simulink model "Dfig"  (R2017b)
settings: Solver=ode45  StartTime=0.0  StopTime=20  RelTol=1e-3  EnableMultiTasking=on
undefined symbols (not defined in the file): Cbus, D, DiscIntNeverNeededParam, f, Fs, fsw, J, ki_id, ki_n, kp_id, kp_n, Lg, Lm, Lr, Ls, Lsi, p, Ps, Rg, Rr, Rs, sigma, Tem, Ts, Vbus, Vs
libraries: powerlib x15, powerlib_meascontrol x2
settings Model: Creator=admin  LastModifiedBy=admin
settings DataIOCC: LimitDataPoints=on  SaveFormat=Array
settings OptimizationCC: LifeSpan=inf
settings DebuggingCC: UnderspecifiedInitializationDetection=Classic  MergeDetectMultiDrivingBlocksExec=none  SolverPrmCheckMsg=warning  StateNameClashWarn=warning  SFUnexpectedBacktrackingDiag=warning  SFNoUnconditionalDefaultTransitionDiag=warning  SFExecutionAtInitializationDiag=none
settings HardwareCC: ProdBitPerPointer=32  ProdBitPerSizeT=32  ProdBitPerPtrDiffT=32  ProdLargestAtomicFloat=None  ProdIntDivRoundTo=Undefined  ProdEndianess=Unspecified  ProdWordSize=32  ProdHWDeviceType=32-bit Generic
settings ModelReferenceCC: PropagateSignalLabelsOutOfModel=off
settings CodeAppCC: StateflowObjectComments=on
settings GRTTargetCC: TargetLangStandard=C89/C90 (ANSI)  GeneratePreprocessorConditionals=Disable all
settings ConfigComp: CovMetricSettings=dw  CovHtmlReporting=on  CovSaveCumulativeToWorkspaceVar=on  CovSaveSingleToWorkspaceVar=on  CovExternalEMLEnable=off
settings SimscapeCC: SimscapeNormalizeSystem=off

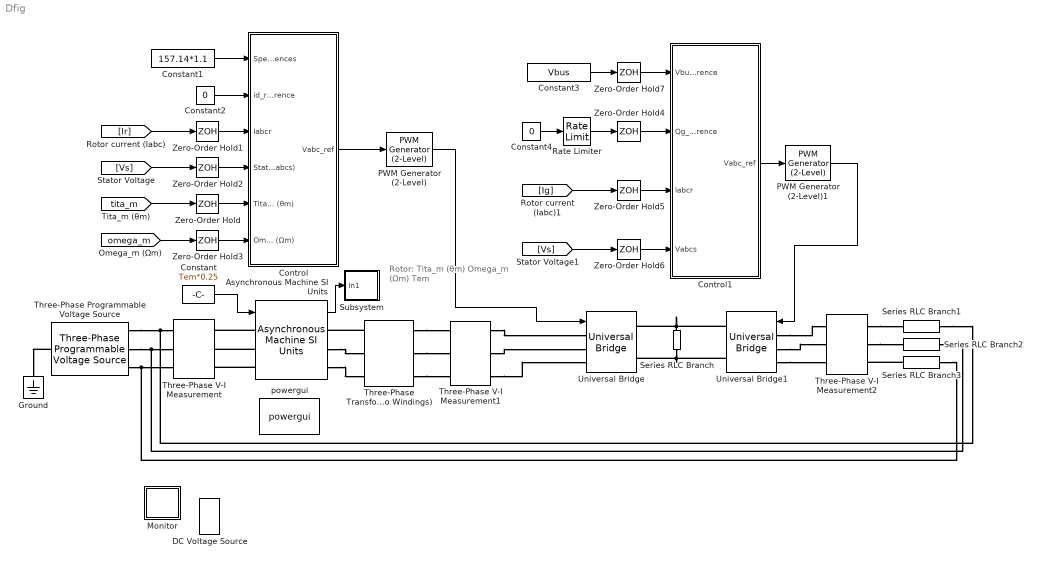
== system Dfig ==
  note: Rotor:
      | Tita_m (θm)
      | Omega_m (Ωm)
      | Tem
  Asynchronous Machine SI Units : powerlib/Machines/Asynchronous Machine SI Units  RotorType=Wound  PresetModel=No  MechanicalLoad=Torque Tm  ShowDetailedParameters=on  ReferenceFrame=Rotor  Units=SI  MeasurementBus=off  NominalParameters=[ Ps Vs f ]  Stator=[ Rs , Lsi]  Rotor=[ Rr , Lsi]  Cage1=[ 0.022 0.226/377]  Cage2=[ 0.022 0.226/377]  Lm=Lm  Mechanical=[ J D 2 ]  PolePairs=2  InitialConditions=[1 0 0 0 0 0 0 0]  SimulateSaturation=off  Saturation=[14.03593122, 27.81365428, 53.79336849, 72.68890987, 97.98006896, 148.6815601, 215.7428561, 302.9841135, 420.4778367 ; 230, 322, 414, 460, 506, 552, 598, 644, 690]  LoadFlowParameters=1492000  TsPowergui=0  TsBlock=-1  IterativeModel=Trapezoidal non iterative  IterativeDiscreteModel=Trapezoidal non iterative  Pmec=0
  Constant : Constant  Value=Tem*0.25
  Constant1 : Constant  Value=157.14*1.1
  Constant2 : Constant  Value=0
  Constant3 : Constant  Value=Vbus
  Constant4 : Constant  Value=0
  Control : Subsystem
  Control1 : Subsystem
  DC Voltage Source : powerlib/Electrical Sources/DC Voltage Source  Amplitude=Vbus  Measurements=None
  Ground : powerlib/Elements/Ground  LConnTagsString=a
  Monitor : Subsystem
  PWM Generator (2-Level) : powerlib_meascontrol/Pulse & Signal Generators/PWM Generator (2-Level)  ModulatorType=Three-phase bridge (6 pulses)  ModulatorMode=Unsynchronized  Fc=fsw  Pc=0  nF=27  MinMax="[ -1  1 ]"  SamplingTechnique=Natural  ModulatingSignals=off  m=0.8  Freq=60  Phase=0  Ts=0  ShowCarrierOutport=off
      settings: SourceProductName=Simscape Power Systems
  PWM Generator (2-Level)1 : powerlib_meascontrol/Pulse & Signal Generators/PWM Generator (2-Level)  ModulatorType=Three-phase bridge (6 pulses)  ModulatorMode=Unsynchronized  Fc=fsw  Pc=0  nF=27  MinMax="[ -1  1 ]"  SamplingTechnique=Natural  ModulatingSignals=off  m=0.8  Freq=60  Phase=0  Ts=0  ShowCarrierOutport=off
      settings: SourceProductName=Simscape Power Systems
  Rate Limiter : RateLimiter  RisingSlewLimit=1000e3/2  FallingSlewLimit=-1000e3/2  SampleTimeMode=inherited
  Series RLC Branch : powerlib/Elements/Series RLC Branch  LConnTagsString=__new0  RConnTagsString=__new0  BranchType=C  Resistance=1  Inductance=1e-3  SetiL0=off  InitialCurrent=0  Capacitance=Cbus  Setx0=on  InitialVoltage=0  Measurements=Branch voltage
  Series RLC Branch1 : powerlib/Elements/Series RLC Branch  LConnTagsString=__new0  RConnTagsString=__new0  BranchType=RL  Resistance=Rg  Inductance=Lg  SetiL0=off  InitialCurrent=0  Capacitance=Cbus  Setx0=on  InitialVoltage=0  Measurements=None
  Series RLC Branch2 : powerlib/Elements/Series RLC Branch  LConnTagsString=__new0  RConnTagsString=__new0  BranchType=RL  Resistance=Rg  Inductance=Lg  SetiL0=off  InitialCurrent=0  Capacitance=Cbus  Setx0=on  InitialVoltage=0  Measurements=None
  Series RLC Branch3 : powerlib/Elements/Series RLC Branch  LConnTagsString=__new0  RConnTagsString=__new0  BranchType=RL  Resistance=Rg  Inductance=Lg  SetiL0=off  InitialCurrent=0  Capacitance=Cbus  Setx0=on  InitialVoltage=0  Measurements=None
  Subsystem : Subsystem
  Three-Phase Programmable Voltage Source : powerlib/Electrical Sources/Three-Phase Programmable Voltage Source  PositiveSequence="[Vs  0 f]"  VariationEntity=None  VariationType=Table of time-amplitude pairs  VariationTypeAlt=Step  VariationStep=0.5  VariationRate=10  VariationMagnitude=0.3  VariationFrequency=2  VariationTiming=[1 2]  VariationPhaseA=off  Amplitudes=[1 0.8 1.2 1.0]  TimeValues=[0 0.1 0.15 0.2]  HarmonicGeneration=off  HarmonicA=[3 0.2 -25 0]  HarmonicB=[2 0.15 35 2]  Timing="[0.05  3]"  BusType=swing  Pref=0  Qref=0  Qmin=-inf  Qmax=inf
  Three-Phase Transformer (Two Windings) : powerlib/Elements/Three-Phase Transformer (Two Windings)  Winding1Connection=Y  Winding2Connection=Y  CoreType=Three single-phase transformers  SetSaturation=off  Hysteresis=off  DataFile='hysteresis'  SetInitialFlux=off  Measurements=None  UNITS=SI  NominalPower=[ Ps , f ]  Winding1=[Vs 0 0]  Winding2=[Vs/u 0 0]  Rm=1.0805e+06  Lm=2866  L0=0.5  Saturation=[0 0;0.66653 1910.3;277.72 2419.7]  InitialFluxes=[1273.5 -1273.5 1114.3]  MoreParameters=off  BreakLoop=off  DataType=on  TransfoNumber=1
  Three-Phase V-I Measurement : powerlib/Measurements/Three-Phase V-I Measurement  VoltageMeasurement=phase-to-ground  SetLabelV=on  LabelV=Vs  Vpu=off  VpuLL=off  CurrentMeasurement=yes  SetLabelI=on  LabelI=Is  Ipu=off  Pbase=100e6  Vbase=500e3  OutputType=Complex  PhasorSimulation=off  PSBequivalent=0
  Three-Phase V-I Measurement1 : powerlib/Measurements/Three-Phase V-I Measurement  VoltageMeasurement=phase-to-phase  SetLabelV=on  LabelV=Vr  Vpu=off  VpuLL=off  CurrentMeasurement=yes  SetLabelI=on  LabelI=Ir  Ipu=off  Pbase=100e6  Vbase=500e3  OutputType=Complex  PhasorSimulation=off  PSBequivalent=0
  Three-Phase V-I Measurement2 : powerlib/Measurements/Three-Phase V-I Measurement  VoltageMeasurement=no  SetLabelV=on  LabelV=Vs  Vpu=off  VpuLL=off  CurrentMeasurement=yes  SetLabelI=on  LabelI=Ig  Ipu=off  Pbase=100e6  Vbase=500e3  OutputType=Complex  PhasorSimulation=off  PSBequivalent=0
  Universal Bridge : powerlib/Power Electronics/Universal Bridge  Arms=3  SnubberResistance=1e5  SnubberCapacitance=inf  Device=Ideal Switches  Ron=1e-3  Lon=0  ForwardVoltages="[  0  0  ]"  ForwardVoltage=0  GTOparameters=[ 10e-6 , 20e-6 ]  IGBTparameters=[ 1e-6 , 2e-6 ]  Measurements=None  Measurements_2=None  converterType=Rectifier
  Universal Bridge1 : powerlib/Power Electronics/Universal Bridge  Arms=3  SnubberResistance=1e5  SnubberCapacitance=inf  Device=Ideal Switches  Ron=1e-3  Lon=0  ForwardVoltages="[  0  0  ]"  ForwardVoltage=0  GTOparameters=[ 10e-6 , 20e-6 ]  IGBTparameters=[ 1e-6 , 2e-6 ]  Measurements=None  Measurements_2=None  converterType=Rectifier
  Zero-Order Hold{,1..7} (8 alike) : ZeroOrderHold  SampleTime=1/fsw
  powergui : powerlib/powergui  Priority=1  SimulationMode=Discrete  SampleTime=Ts  frequency=60  Iterations=50  frequencyindice=50  Pbase=100e6  ErrMax=1e-4  UnitsV=kV  UnitsW=MW  buscounter=0  FunctionMessages=off  echomessages=off  EnableUseOfTLC=off  CurrentSourceSwitches=off  DisableSnubberDevices=off  DisableRonSwitches=off  DisableVfSwitches=off  DisplayEquations=off  SolverType=Tustin  Interpol=off  ExternalGateDelay=off  methode=off  Ts=0  x0status=blocks  SPID=off  SwTol=0  HookPort=off  RestoreLinks=warning  ResistiveCurrentMeasurement=off  Frange=[0:2:500]  Ylog=off  Xlog=on  ShowGrid=off  save=off  variable=ZData  structure=0  ZoomFFT=off  StartTime=0.0  cycles=1  DisplayStyle=1  fundamental=60  FreqAxis=off  MaxFrequency=1000  frequencyindicesteady=1  RmsSteady=1  display=off
  wires:
  Constant/1 -> Asynchronous Machine SI Units/1
  PWM Generator (2-Level)/1 -> Universal Bridge/1
  Control/1(Vabc_ref) -> PWM Generator (2-Level)/1
  Constant1/1 -> Control/1(Speed reference Omega_m (Ωm) references)
  Constant2/1 -> Control/2(id_reference)
  [Vs] -> Zero-Order Hold2/1
  [Ir] -> Zero-Order Hold1/1
  Asynchronous Machine SI Units/1 -> Subsystem/1(In1)
  [tita_m] -> Zero-Order Hold/1
  [omega_m] -> Zero-Order Hold3/1
  Zero-Order Hold1/1 -> Control/3(Iabcr)
  Zero-Order Hold2/1 -> Control/4(Stator Voltage (Vabcs))
  Zero-Order Hold/1 -> Control/5(Tita_m (θm))
  Zero-Order Hold3/1 -> Control/6(Omega_m (Ωm))
  Zero-Order Hold6/1 -> Control1/4(Vabcs)
  Zero-Order Hold5/1 -> Control1/3(Iabcr)
  [Ig] -> Zero-Order Hold5/1
  [Vs] -> Zero-Order Hold6/1
  Constant4/1 -> Rate Limiter/1
  Constant3/1 -> Zero-Order Hold7/1
  Control1/1(Vabc_ref) -> PWM Generator (2-Level)1/1
  PWM Generator (2-Level)1/1 -> Universal Bridge1/1
  Rate Limiter/1 -> Zero-Order Hold4/1
  Zero-Order Hold4/1 -> Control1/2(Qg_reference)
  Zero-Order Hold7/1 -> Control1/1("Vbus_reference ")
  connections:
  Three-Phase Programmable Voltage Source/LConn1 -- Ground/LConn1
  Three-Phase Programmable Voltage Source/RConn1 -- Series RLC Branch1/LConn1 -- Three-Phase V-I Measurement/LConn1
  Three-Phase Programmable Voltage Source/RConn2 -- Series RLC Branch2/LConn1 -- Three-Phase V-I Measurement/LConn2
  Three-Phase Programmable Voltage Source/RConn3 -- Series RLC Branch3/LConn1 -- Three-Phase V-I Measurement/LConn3
  Asynchronous Machine SI Units/LConn1 -- Three-Phase V-I Measurement/RConn1
  Asynchronous Machine SI Units/LConn2 -- Three-Phase V-I Measurement/RConn2
  Asynchronous Machine SI Units/LConn3 -- Three-Phase V-I Measurement/RConn3
  Three-Phase V-I Measurement1/LConn1 -- Universal Bridge/LConn1
  Three-Phase V-I Measurement1/LConn2 -- Universal Bridge/LConn2
  Three-Phase V-I Measurement1/LConn3 -- Universal Bridge/LConn3
  Universal Bridge1/RConn1 -- Series RLC Branch/LConn1 -- Universal Bridge/RConn1
  Universal Bridge1/RConn2 -- Series RLC Branch/RConn1 -- Universal Bridge/RConn2
  Series RLC Branch3/RConn1 -- Three-Phase V-I Measurement2/RConn3
  Three-Phase V-I Measurement2/RConn2 -- Series RLC Branch2/RConn1
  Three-Phase V-I Measurement2/RConn1 -- Series RLC Branch1/RConn1
  Universal Bridge1/LConn1 -- Three-Phase V-I Measurement2/LConn1
  Universal Bridge1/LConn2 -- Three-Phase V-I Measurement2/LConn2
  Universal Bridge1/LConn3 -- Three-Phase V-I Measurement2/LConn3
  Three-Phase Transformer (Two Windings)/RConn1 -- Three-Phase V-I Measurement1/RConn1
  Three-Phase Transformer (Two Windings)/RConn2 -- Three-Phase V-I Measurement1/RConn2
  Three-Phase Transformer (Two Windings)/RConn3 -- Three-Phase V-I Measurement1/RConn3
  Three-Phase Transformer (Two Windings)/LConn1 -- Asynchronous Machine SI Units/RConn1
  Asynchronous Machine SI Units/RConn2 -- Three-Phase Transformer (Two Windings)/LConn2
  Asynchronous Machine SI Units/RConn3 -- Three-Phase Transformer (Two Windings)/LConn3

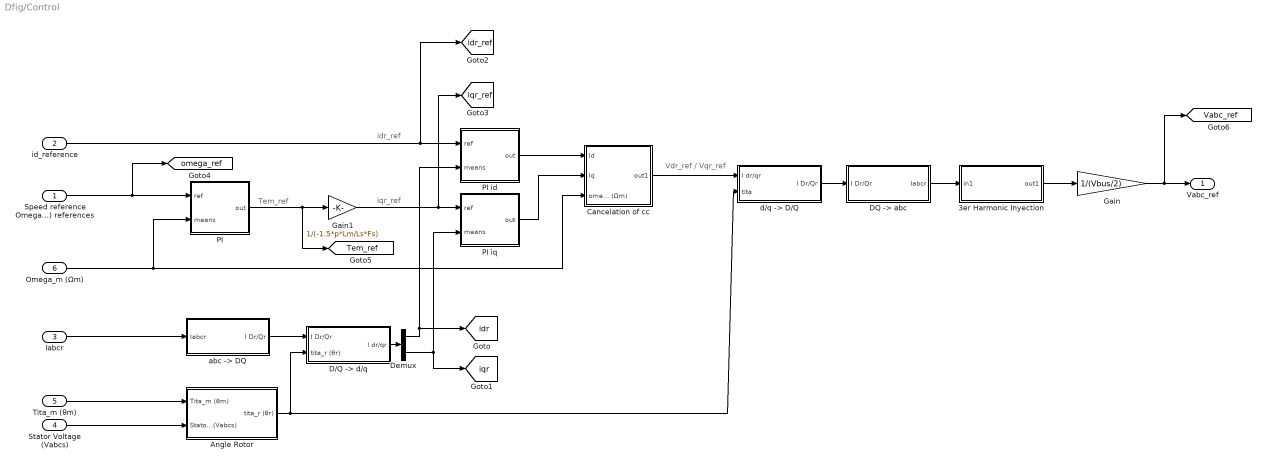
== system Dfig/Control ==
  note: Vdr_ref / Vqr_ref
  note: iqr_ref
  note: Tem_ref
  note: idr_ref
  Speed reference Omega_m (Ωm) references : Inport
  id_reference : Inport  Port=2
  Iabcr : Inport  Port=3
  Stator Voltage (Vabcs) : Inport  Port=4
  Tita_m (θm) : Inport  Port=5
  Omega_m (Ωm) : Inport  Port=6
  " Angle Rotor" : Subsystem
  3er Harmonic Inyection : Subsystem
  Cancelation of cc : Subsystem
  "D/Q -> d/q" : Subsystem
  "DQ -> abc" : Subsystem
  Demux : Demux  Outputs=2
  Gain : Gain  Gain=1/(Vbus/2)
  Gain1 : Gain  Gain=1/(-1.5*p*Lm/Ls*Fs)
  PI : Subsystem
  PI id : Subsystem
  PI iq : Subsystem
  "abc -> DQ " : Subsystem
  "d/q -> D/Q " : Subsystem
  Vabc_ref : Outport
  tag scope: Tem_ref=global, Vabc_ref=global, idr=global, idr_ref=global, iqr=global, iqr_ref=global, omega_ref=global
  wires:
  Gain/1 -> [Vabc_ref], Vabc_ref/1
  "DQ -> abc"/1(Iabcr) -> 3er Harmonic Inyection/1(in1)
  "d/q -> D/Q "/1(I Dr/Qr) -> "DQ -> abc"/1(I Dr/Qr)
  Iabcr/1 -> "abc -> DQ "/1(Iabcr)
  "abc -> DQ "/1(I Dr/Qr) -> "D/Q -> d/q"/1(I Dr/Qr)
  3er Harmonic Inyection/1(out1) -> Gain/1
  Tita_m (θm)/1 -> " Angle Rotor"/1(Tita_m (θm))
  Stator Voltage (Vabcs)/1 -> " Angle Rotor"/2(Stator Voltage (Vabcs))
  " Angle Rotor"/1(tita_r (θr)) -> "D/Q -> d/q"/2(tita_r (θr)), "d/q -> D/Q "/2(tita)
  PI id/1(out) -> Cancelation of cc/1(Id)
  PI iq/1(out) -> Cancelation of cc/2(Iq)
  Omega_m (Ωm)/1 -> PI/2(means), Cancelation of cc/3(omega_m (Ωm))
  "D/Q -> d/q"/1(I dr/qr) -> Demux/1
  Demux/2 -> [iqr], PI iq/2(means)
  Demux/1 -> [idr], PI id/2(means)
  Speed reference Omega_m (Ωm) references/1 -> PI/1(ref), [omega_ref]
  PI/1(out) -> [Tem_ref], Gain1/1
  Gain1/1 -> [iqr_ref], PI iq/1(ref)
  id_reference/1 -> [idr_ref], PI id/1(ref)
  Cancelation of cc/1(out1) -> "d/q -> D/Q "/1(I dr/qr)

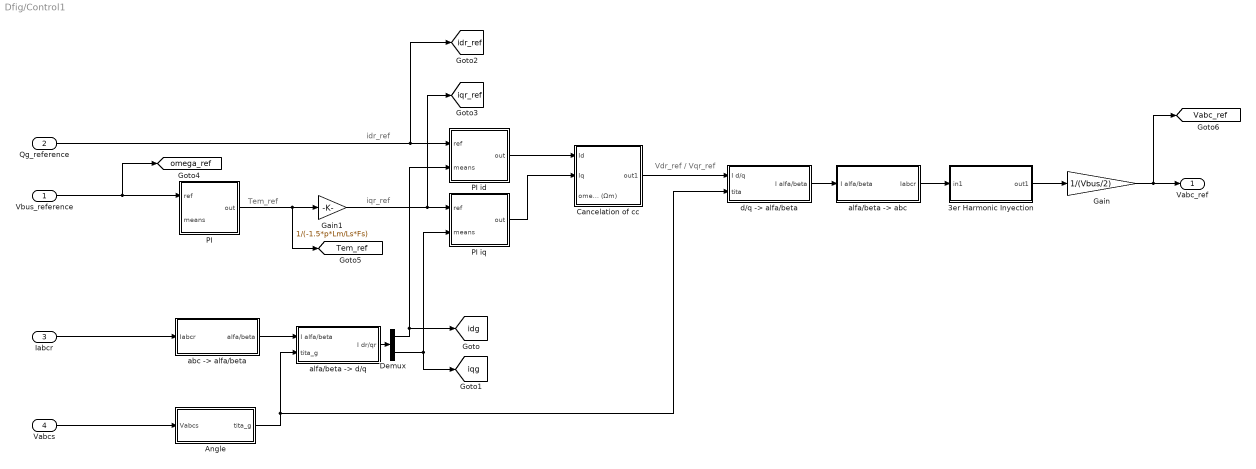
== system Dfig/Control1 ==
  note: idr_ref
  note: Tem_ref
  note: iqr_ref
  note: Vdr_ref / Vqr_ref
  "Vbus_reference " : Inport
  Qg_reference : Inport  Port=2
  Iabcr : Inport  Port=3
  Vabcs : Inport  Port=4
  " Angle" : Subsystem
  3er Harmonic Inyection : Subsystem
  Cancelation of cc : Subsystem
  Demux : Demux  Outputs=2
  Gain : Gain  Gain=1/(Vbus/2)
  Gain1 : Gain  Gain=1/(-1.5*p*Lm/Ls*Fs)
  PI : Subsystem
  PI id : Subsystem
  PI iq : Subsystem
  "abc -> alfa/beta " : Subsystem
  "alfa/beta -> abc" : Subsystem
  "alfa/beta -> d/q" : Subsystem
  "d/q -> alfa/beta " : Subsystem
  Vabc_ref : Outport
  tag scope: Tem_ref=global, Vabc_ref=global, idg=global, idr_ref=global, iqg=global, iqr_ref=global, omega_ref=global
  wires:
  Cancelation of cc/1(out1) -> "d/q -> alfa/beta "/1(I d/q)
  Qg_reference/1 -> PI id/1(ref), [idr_ref]
  Gain1/1 -> PI iq/1(ref), [iqr_ref]
  PI/1(out) -> Gain1/1, [Tem_ref]
  "Vbus_reference "/1 -> [omega_ref], PI/1(ref)
  Demux/1 -> PI id/2(means), [idg]
  Demux/2 -> PI iq/2(means), [iqg]
  "alfa/beta -> d/q"/1(I dr/qr) -> Demux/1
  PI iq/1(out) -> Cancelation of cc/2(Iq)
  PI id/1(out) -> Cancelation of cc/1(Id)
  " Angle"/1(tita_g) -> "d/q -> alfa/beta "/2(tita), "alfa/beta -> d/q"/2(tita_g)
  Vabcs/1 -> " Angle"/1(Vabcs)
  3er Harmonic Inyection/1(out1) -> Gain/1
  "abc -> alfa/beta "/1(alfa/beta) -> "alfa/beta -> d/q"/1(I alfa/beta)
  Iabcr/1 -> "abc -> alfa/beta "/1(Iabcr)
  "d/q -> alfa/beta "/1(I alfa/beta) -> "alfa/beta -> abc"/1(I alfa/beta)
  "alfa/beta -> abc"/1(Iabcr) -> 3er Harmonic Inyection/1(in1)
  Gain/1 -> Vabc_ref/1, [Vabc_ref]

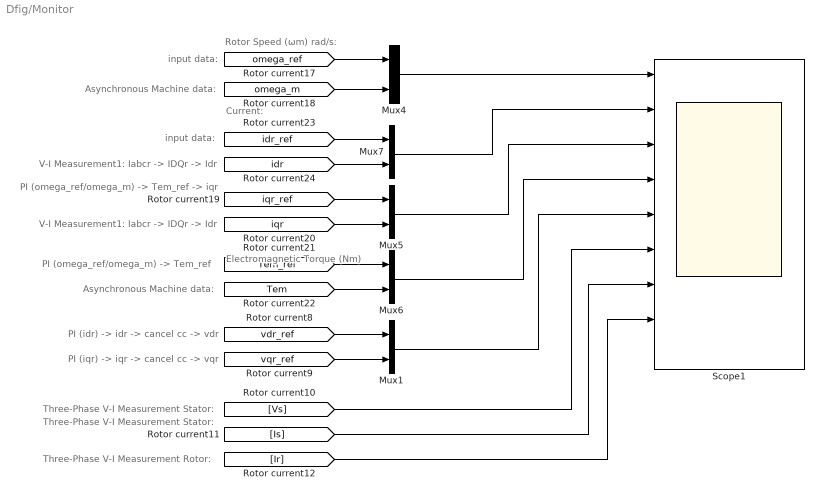
== system Dfig/Monitor ==
  note: Electromagnetic Torque (Nm)
  note: Three-Phase V-I Measurement Stator:
  note: PI (idr) -> idr -> cancel cc -> vdr
  note: PI (omega_ref/omega_m) -> Tem_ref -> iqr
  note: V-I Measurement1: Iabcr -> IDQr -> Idr
  note: input data:
  note: Current:
  note: Rotor Speed (ωm) rad/s:
  note: Asynchronous Machine data:
  note: input data:
  note: V-I Measurement1: Iabcr -> IDQr -> Idr
  note: PI (omega_ref/omega_m) -> Tem_ref
  note: Asynchronous Machine data:
  note: PI (iqr) -> iqr -> cancel cc -> vqr
  note: Three-Phase V-I Measurement Stator:
  note: Three-Phase V-I Measurement Rotor:
  Mux{1,4..7} (5 alike) : Mux  Inputs=2
  Scope1 : Scope  NumInputPorts=9
  wires:
  [omega_m] -> Mux4/2
  [omega_ref] -> Mux4/1
  [iqr_ref] -> Mux5/1
  [iqr] -> Mux5/2
  [Tem] -> Mux6/2
  [Tem_ref] -> Mux6/1
  [idr] -> Mux7/2
  [idr_ref] -> Mux7/1
  Mux4/1 -> Scope1/1
  [vdr_ref] -> Mux1/1
  [vqr_ref] -> Mux1/2
  Mux7/1 -> Scope1/2
  Mux5/1 -> Scope1/3
  Mux6/1 -> Scope1/4
  Mux1/1 -> Scope1/5
  [Vs] -> Scope1/6
  [Is] -> Scope1/7
  [Ir] -> Scope1/8

== system Dfig/Subsystem ==
  In1 : Inport
  Bus Selector : BusSelector  OutputSignals=Mechanical.Rotor angle thetam (rad),Mechanical.Rotor speed (wm),Mechanical.Electromagnetic torque Te (N*m)
  Scope : Scope  NumInputPorts=3
  tag scope: Tem=global, omega_m=global, tita_m=global
  wires:
  Bus Selector/2 -> Scope/2, [omega_m]  "<Rotor speed (wm)>"
  In1/1 -> Bus Selector/1
  Bus Selector/1 -> Scope/1, [tita_m]  "<Rotor angle thetam (rad)>"
  Bus Selector/3 -> Scope/3, [Tem]  "<Electromagnetic torque Te (N*m)>"

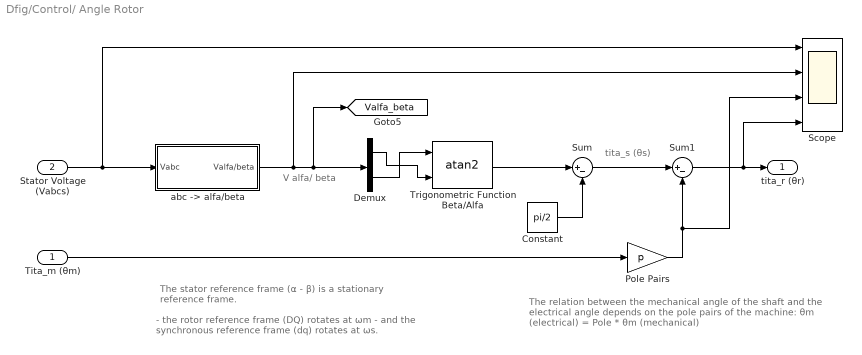
== system Dfig/Control/ Angle Rotor ==
  note: - the rotor reference frame (DQ) rotates at ωm
      | - and the synchronous reference frame (dq) rotates at ωs.
  note: The stator reference frame (α - β) is a stationary
      | reference frame.
  note: The relation between the mechanical angle of the shaft  and the
      | electrical angle depends on the pole pairs of the machine:
      |
      | θm (electrical) = Pole * θm (mechanical)
  note: tita_s (θs)
  note: V alfa/ beta
  Tita_m (θm) : Inport
  Stator Voltage (Vabcs) : Inport  Port=2
  Constant : Constant  Value=pi/2
  Demux : Demux  Outputs=2
  Pole Pairs : Gain  Gain=p
  Scope : Scope  NumInputPorts=4
  Sum : Sum  Inputs=|+-
  Sum1 : Sum  Inputs=|+-
  Trigonometric Function Beta/Alfa : Trigonometry  Operator=atan2
  "abc -> alfa/beta " : Subsystem
  tita_r (θr) : Outport
  tag scope: Valfa_beta=global
  wires:
  Stator Voltage (Vabcs)/1 -> Scope/1, "abc -> alfa/beta "/1(Vabc)
  Demux/2 -> Trigonometric Function Beta/Alfa/1
  Demux/1 -> Trigonometric Function Beta/Alfa/2
  "abc -> alfa/beta "/1("Valfa/beta ") -> Scope/2, [Valfa_beta], Demux/1
  Trigonometric Function Beta/Alfa/1 -> Sum/1
  Constant/1 -> Sum/2
  Tita_m (θm)/1 -> Pole Pairs/1
  Sum/1 -> Sum1/1
  Sum1/1 -> Scope/4, tita_r (θr)/1
  Pole Pairs/1 -> Sum1/2, Scope/3

== system Dfig/Control/3er Harmonic Inyection ==
  in1 : Inport
  Gain : Gain  Gain=-0.5
  MinMax : MinMax
  MinMax1 : MinMax  Function=max
  Sum : Sum  Inputs=|++
  Sum1 : Sum  Inputs=|++
  out1 : Outport
  wires:
  in1/1 -> Sum1/1, MinMax1/1, MinMax/1
  MinMax/1 -> Sum/1
  MinMax1/1 -> Sum/2
  Sum1/1 -> out1/1
  Sum/1 -> Gain/1
  Gain/1 -> Sum1/2

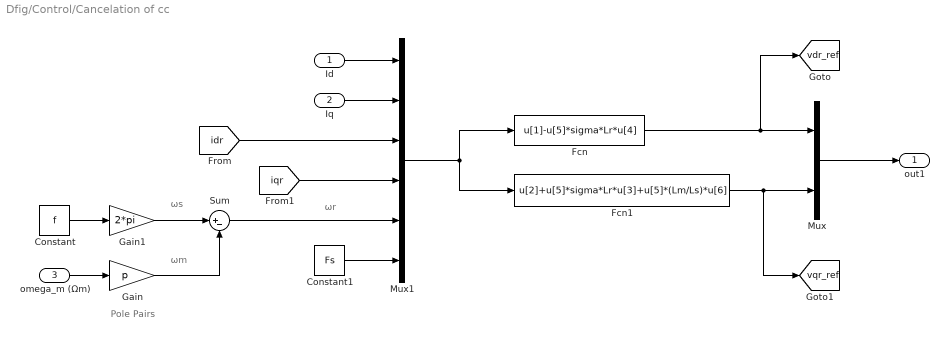
== system Dfig/Control/Cancelation of cc ==
  note: Pole Pairs
  note: ωr
  note: ωm
  note: ωs
  Id : Inport
  Iq : Inport  Port=2
  omega_m (Ωm) : Inport  Port=3
  Constant : Constant  Value=f
  Constant1 : Constant  Value=Fs
  Fcn : Fcn  Expr=u[1]-u[5]*sigma*Lr*u[4]
  Fcn1 : Fcn  Expr=u[2]+u[5]*sigma*Lr*u[3]+u[5]*(Lm/Ls)*u[6]
  Gain : Gain  Gain=p
  Gain1 : Gain  Gain=2*pi
  Mux : Mux  Inputs=2
  Mux1 : Mux  Inputs=6
  Sum : Sum  Inputs=|+-
  out1 : Outport
  tag scope: vdr_ref=global, vqr_ref=global
  wires:
  Mux/1 -> out1/1
  Fcn/1 -> [vdr_ref], Mux/1
  Fcn1/1 -> [vqr_ref], Mux/2
  Id/1 -> Mux1/1
  Iq/1 -> Mux1/2
  Mux1/1 -> Fcn1/1, Fcn/1
  [idr] -> Mux1/3
  [iqr] -> Mux1/4
  Constant1/1 -> Mux1/6
  omega_m (Ωm)/1 -> Gain/1
  Gain/1 -> Sum/2
  Constant/1 -> Gain1/1
  Gain1/1 -> Sum/1
  Sum/1 -> Mux1/5

== system Dfig/Control/D//Q -> d//q ==
  I Dr/Qr : Inport
  tita_r (θr) : Inport  Port=2
  Fcn : Fcn  Expr=u(1)*cos(u[3])+u[2]*sin(u[3])
  Fcn1 : Fcn  Expr=-u(1)*sin(u[3])+u[2]*cos(u[3])
  Mux : Mux  Inputs=2
  Mux1 : Mux  Inputs=2
  Scope : Scope  NumInputPorts=3
  I dr/qr : Outport
  wires:
  Mux/1 -> Scope/3, I dr/qr/1
  Fcn/1 -> Mux/1
  Fcn1/1 -> Mux/2
  I Dr/Qr/1 -> Scope/1, Mux1/1
  tita_r (θr)/1 -> Scope/2, Mux1/2
  Mux1/1 -> Fcn/1, Fcn1/1

== system Dfig/Control/DQ -> abc ==
  I Dr/Qr : Inport
  Fcn : Fcn  Expr=u(1)
  Fcn1 : Fcn  Expr=-(u[1]/2)+u[2]*(sqrt(3)/2)
  Fcn2 : Fcn  Expr=-(u[1]/2)-u[2]*(sqrt(3)/2)
  Mux : Mux  Inputs=3
  Iabcr : Outport
  wires:
  Mux/1 -> Iabcr/1
  I Dr/Qr/1 -> Fcn2/1, Fcn1/1, Fcn/1
  Fcn/1 -> Mux/1
  Fcn1/1 -> Mux/2
  Fcn2/1 -> Mux/3

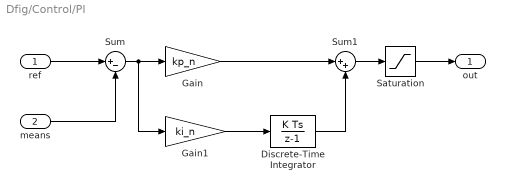
== system Dfig/Control/PI ==
  ref : Inport
  means : Inport  Port=2
  Discrete-Time Integrator : DiscreteIntegrator  SampleTime=1/fsw  LimitOutput=on  UpperSaturationLimit=Tem  LowerSaturationLimit=-Tem  ICPrevOutput=DiscIntNeverNeededParam  ICPrevScaledInput=DiscIntNeverNeededParam
  Gain : Gain  Gain=kp_n
  Gain1 : Gain  Gain=ki_n
  Saturation : Saturate  UpperLimit=Tem  LowerLimit=-Tem
  Sum : Sum  Inputs=|+-
  Sum1 : Sum  Inputs=|++
  out : Outport
  wires:
  means/1 -> Sum/2
  ref/1 -> Sum/1
  Sum/1 -> Gain1/1, Gain/1
  Gain/1 -> Sum1/1
  Gain1/1 -> Discrete-Time Integrator/1
  Discrete-Time Integrator/1 -> Sum1/2
  Sum1/1 -> Saturation/1
  Saturation/1 -> out/1

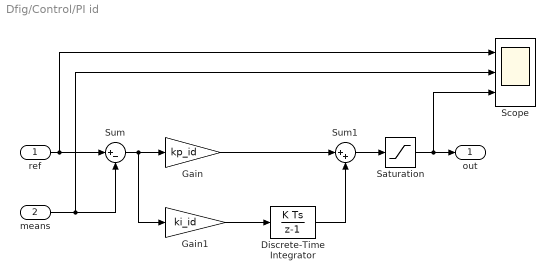
== system Dfig/Control/PI id ==
  ref : Inport
  means : Inport  Port=2
  Discrete-Time Integrator : DiscreteIntegrator  SampleTime=1/fsw  LimitOutput=on  UpperSaturationLimit=Vbus/sqrt(3)  LowerSaturationLimit=-Vbus/sqrt(3)  ICPrevOutput=DiscIntNeverNeededParam  ICPrevScaledInput=DiscIntNeverNeededParam
  Gain : Gain  Gain=kp_id
  Gain1 : Gain  Gain=ki_id
  Saturation : Saturate  UpperLimit=Vbus/sqrt(3)  LowerLimit=-Vbus/sqrt(3)
  Scope : Scope  NumInputPorts=3
  Sum : Sum  Inputs=|+-
  Sum1 : Sum  Inputs=|++
  out : Outport
  wires:
  means/1 -> Scope/2, Sum/2
  ref/1 -> Scope/1, Sum/1
  Sum/1 -> Gain1/1, Gain/1
  Gain/1 -> Sum1/1
  Gain1/1 -> Discrete-Time Integrator/1
  Discrete-Time Integrator/1 -> Sum1/2
  Sum1/1 -> Saturation/1
  Saturation/1 -> Scope/3, out/1

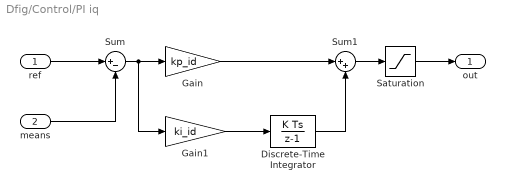
== system Dfig/Control/PI iq ==
  ref : Inport
  means : Inport  Port=2
  Discrete-Time Integrator : DiscreteIntegrator  SampleTime=1/fsw  LimitOutput=on  UpperSaturationLimit=Vbus/sqrt(3)  LowerSaturationLimit=-Vbus/sqrt(3)  ICPrevOutput=DiscIntNeverNeededParam  ICPrevScaledInput=DiscIntNeverNeededParam
  Gain : Gain  Gain=kp_id
  Gain1 : Gain  Gain=ki_id
  Saturation : Saturate  UpperLimit=Vbus/sqrt(3)  LowerLimit=-Vbus/sqrt(3)
  Sum : Sum  Inputs=|+-
  Sum1 : Sum  Inputs=|++
  out : Outport
  wires:
  means/1 -> Sum/2
  ref/1 -> Sum/1
  Sum/1 -> Gain1/1, Gain/1
  Gain/1 -> Sum1/1
  Gain1/1 -> Discrete-Time Integrator/1
  Discrete-Time Integrator/1 -> Sum1/2
  Sum1/1 -> Saturation/1
  Saturation/1 -> out/1

== system Dfig/Control/abc -> DQ  ==
  note: IQr
  note: IDr
  Iabcr : Inport
  Fcn : Fcn  Expr=2/3*(u[1]-u[2]/2-u[3]/2)
  Fcn1 : Fcn  Expr=2/3*(u[2]*(sqrt(3)/2)-u[3]*(sqrt(3)/2))
  Mux : Mux  Inputs=2
  Scope : Scope  NumInputPorts=2
  I Dr/Qr : Outport
  wires:
  Mux/1 -> Scope/2, I Dr/Qr/1
  Iabcr/1 -> Scope/1, Fcn1/1, Fcn/1
  Fcn/1 -> Mux/1
  Fcn1/1 -> Mux/2

== system Dfig/Control/d//q -> D//Q  ==
  I dr/qr : Inport
  tita : Inport  Port=2
  Fcn : Fcn  Expr=u(1)*cos(u[3])-u[2]*sin(u[3])
  Fcn1 : Fcn  Expr=u(1)*sin(u[3])+u[2]*cos(u[3])
  Mux : Mux  Inputs=2
  Mux1 : Mux  Inputs=2
  I Dr/Qr : Outport
  wires:
  Mux/1 -> I Dr/Qr/1
  Fcn/1 -> Mux/1
  Fcn1/1 -> Mux/2
  I dr/qr/1 -> Mux1/1
  tita/1 -> Mux1/2
  Mux1/1 -> Fcn/1, Fcn1/1

== system Dfig/Control1/ Angle ==
  note: tita_g
  note: V alfa/ beta
  Vabcs : Inport
  Demux : Demux  Outputs=2
  Trigonometric Function Beta/Alfa : Trigonometry  Operator=atan2
  "abc -> alfa/beta " : Subsystem
  tita_g : Outport
  wires:
  "abc -> alfa/beta "/1("Valfa/beta ") -> Demux/1
  Demux/1 -> Trigonometric Function Beta/Alfa/2
  Demux/2 -> Trigonometric Function Beta/Alfa/1
  Vabcs/1 -> "abc -> alfa/beta "/1(Vabc)
  Trigonometric Function Beta/Alfa/1 -> tita_g/1

== system Dfig/Control1/3er Harmonic Inyection ==
  in1 : Inport
  Gain : Gain  Gain=-0.5
  MinMax : MinMax
  MinMax1 : MinMax  Function=max
  Sum : Sum  Inputs=|++
  Sum1 : Sum  Inputs=|++
  out1 : Outport
  wires:
  Gain/1 -> Sum1/2
  Sum/1 -> Gain/1
  Sum1/1 -> out1/1
  MinMax1/1 -> Sum/2
  MinMax/1 -> Sum/1
  in1/1 -> MinMax/1, MinMax1/1, Sum1/1

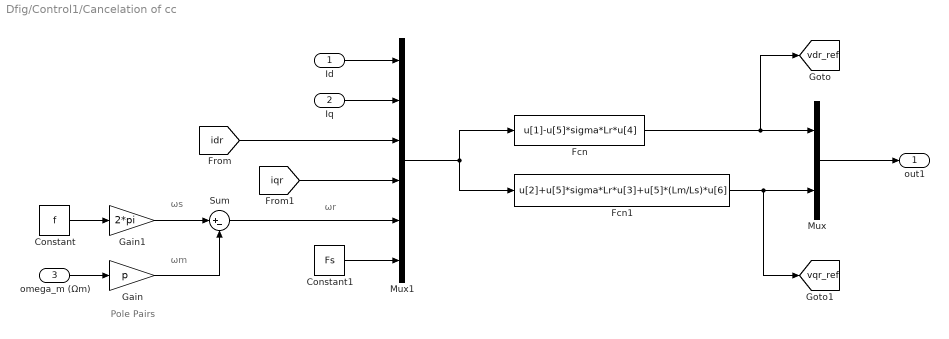
== system Dfig/Control1/Cancelation of cc ==
  note: ωs
  note: ωm
  note: ωr
  note: Pole Pairs
  Id : Inport
  Iq : Inport  Port=2
  omega_m (Ωm) : Inport  Port=3
  Constant : Constant  Value=f
  Constant1 : Constant  Value=Fs
  Fcn : Fcn  Expr=u[1]-u[5]*sigma*Lr*u[4]
  Fcn1 : Fcn  Expr=u[2]+u[5]*sigma*Lr*u[3]+u[5]*(Lm/Ls)*u[6]
  Gain : Gain  Gain=p
  Gain1 : Gain  Gain=2*pi
  Mux : Mux  Inputs=2
  Mux1 : Mux  Inputs=6
  Sum : Sum  Inputs=|+-
  out1 : Outport
  tag scope: vdr_ref=global, vqr_ref=global
  wires:
  Sum/1 -> Mux1/5
  Gain1/1 -> Sum/1
  Constant/1 -> Gain1/1
  Gain/1 -> Sum/2
  omega_m (Ωm)/1 -> Gain/1
  Constant1/1 -> Mux1/6
  [iqr] -> Mux1/4
  [idr] -> Mux1/3
  Mux1/1 -> Fcn/1, Fcn1/1
  Iq/1 -> Mux1/2
  Id/1 -> Mux1/1
  Fcn1/1 -> Mux/2, [vqr_ref]
  Fcn/1 -> Mux/1, [vdr_ref]
  Mux/1 -> out1/1

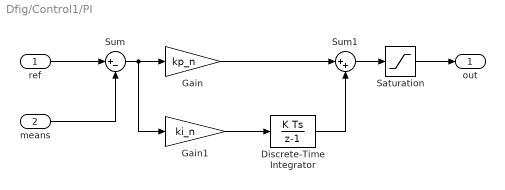
== system Dfig/Control1/PI ==
  ref : Inport
  means : Inport  Port=2
  Discrete-Time Integrator : DiscreteIntegrator  SampleTime=1/fsw  LimitOutput=on  UpperSaturationLimit=Tem  LowerSaturationLimit=-Tem  ICPrevOutput=DiscIntNeverNeededParam  ICPrevScaledInput=DiscIntNeverNeededParam
  Gain : Gain  Gain=kp_n
  Gain1 : Gain  Gain=ki_n
  Saturation : Saturate  UpperLimit=Tem  LowerLimit=-Tem
  Sum : Sum  Inputs=|+-
  Sum1 : Sum  Inputs=|++
  out : Outport
  wires:
  Saturation/1 -> out/1
  Sum1/1 -> Saturation/1
  Discrete-Time Integrator/1 -> Sum1/2
  Gain1/1 -> Discrete-Time Integrator/1
  Gain/1 -> Sum1/1
  Sum/1 -> Gain/1, Gain1/1
  ref/1 -> Sum/1
  means/1 -> Sum/2

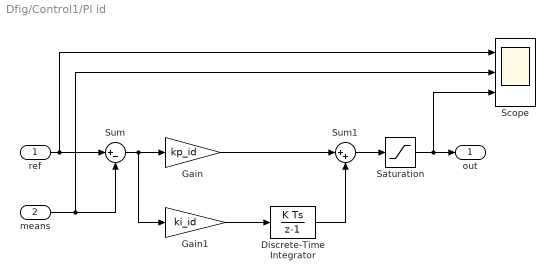
== system Dfig/Control1/PI id ==
  ref : Inport
  means : Inport  Port=2
  Discrete-Time Integrator : DiscreteIntegrator  SampleTime=1/fsw  LimitOutput=on  UpperSaturationLimit=Vbus/sqrt(3)  LowerSaturationLimit=-Vbus/sqrt(3)  ICPrevOutput=DiscIntNeverNeededParam  ICPrevScaledInput=DiscIntNeverNeededParam
  Gain : Gain  Gain=kp_id
  Gain1 : Gain  Gain=ki_id
  Saturation : Saturate  UpperLimit=Vbus/sqrt(3)  LowerLimit=-Vbus/sqrt(3)
  Scope : Scope  NumInputPorts=3
  Sum : Sum  Inputs=|+-
  Sum1 : Sum  Inputs=|++
  out : Outport
  wires:
  Saturation/1 -> out/1, Scope/3
  Sum1/1 -> Saturation/1
  Discrete-Time Integrator/1 -> Sum1/2
  Gain1/1 -> Discrete-Time Integrator/1
  Gain/1 -> Sum1/1
  Sum/1 -> Gain/1, Gain1/1
  ref/1 -> Sum/1, Scope/1
  means/1 -> Sum/2, Scope/2

== system Dfig/Control1/PI iq ==
  ref : Inport
  means : Inport  Port=2
  Discrete-Time Integrator : DiscreteIntegrator  SampleTime=1/fsw  LimitOutput=on  UpperSaturationLimit=Vbus/sqrt(3)  LowerSaturationLimit=-Vbus/sqrt(3)  ICPrevOutput=DiscIntNeverNeededParam  ICPrevScaledInput=DiscIntNeverNeededParam
  Gain : Gain  Gain=kp_id
  Gain1 : Gain  Gain=ki_id
  Saturation : Saturate  UpperLimit=Vbus/sqrt(3)  LowerLimit=-Vbus/sqrt(3)
  Sum : Sum  Inputs=|+-
  Sum1 : Sum  Inputs=|++
  out : Outport
  wires:
  Saturation/1 -> out/1
  Sum1/1 -> Saturation/1
  Discrete-Time Integrator/1 -> Sum1/2
  Gain1/1 -> Discrete-Time Integrator/1
  Gain/1 -> Sum1/1
  Sum/1 -> Gain/1, Gain1/1
  ref/1 -> Sum/1
  means/1 -> Sum/2

== system Dfig/Control1/abc -> alfa//beta  ==
  note: IDr
  note: IQr
  Iabcr : Inport
  Fcn : Fcn  Expr=2/3*(u[1]-u[2]/2-u[3]/2)
  Fcn1 : Fcn  Expr=2/3*(u[2]*(sqrt(3)/2)-u[3]*(sqrt(3)/2))
  Mux : Mux  Inputs=2
  alfa/beta : Outport
  wires:
  Fcn1/1 -> Mux/2
  Fcn/1 -> Mux/1
  Iabcr/1 -> Fcn/1, Fcn1/1
  Mux/1 -> alfa/beta/1

== system Dfig/Control1/alfa//beta -> abc ==
  I alfa/beta : Inport
  Fcn : Fcn  Expr=u(1)
  Fcn1 : Fcn  Expr=-(u[1]/2)+u[2]*(sqrt(3)/2)
  Fcn2 : Fcn  Expr=-(u[1]/2)-u[2]*(sqrt(3)/2)
  Mux : Mux  Inputs=3
  Iabcr : Outport
  wires:
  Fcn2/1 -> Mux/3
  Fcn1/1 -> Mux/2
  Fcn/1 -> Mux/1
  I alfa/beta/1 -> Fcn/1, Fcn1/1, Fcn2/1
  Mux/1 -> Iabcr/1

== system Dfig/Control1/alfa//beta -> d//q ==
  I alfa/beta : Inport
  tita_g : Inport  Port=2
  Fcn : Fcn  Expr=u(1)*cos(u[3])+u[2]*sin(u[3])
  Fcn1 : Fcn  Expr=-u(1)*sin(u[3])+u[2]*cos(u[3])
  Mux : Mux  Inputs=2
  Mux1 : Mux  Inputs=2
  Scope : Scope  NumInputPorts=3
  I dr/qr : Outport
  wires:
  Mux1/1 -> Fcn1/1, Fcn/1
  tita_g/1 -> Mux1/2, Scope/2
  I alfa/beta/1 -> Mux1/1, Scope/1
  Fcn1/1 -> Mux/2
  Fcn/1 -> Mux/1
  Mux/1 -> I dr/qr/1, Scope/3

== system Dfig/Control1/d//q -> alfa//beta  ==
  I d/q : Inport
  tita : Inport  Port=2
  Fcn : Fcn  Expr=u(1)*cos(u[3])-u[2]*sin(u[3])
  Fcn1 : Fcn  Expr=u(1)*sin(u[3])+u[2]*cos(u[3])
  Mux : Mux  Inputs=2
  Mux1 : Mux  Inputs=2
  I alfa/beta : Outport
  wires:
  Mux1/1 -> Fcn1/1, Fcn/1
  tita/1 -> Mux1/2
  I d/q/1 -> Mux1/1
  Fcn1/1 -> Mux/2
  Fcn/1 -> Mux/1
  Mux/1 -> I alfa/beta/1

== system Dfig/Control/ Angle Rotor/abc -> alfa//beta  ==
  Vabc : Inport
  Fcn : Fcn  Expr=2/3*(u[1]-u[2]/2-u[3]/2)
  Fcn1 : Fcn  Expr=2/3*(u[2]*(sqrt(3)/2)-u[3]*(sqrt(3)/2))
  Mux : Mux  Inputs=2
  "Valfa/beta " : Outport
  wires:
  Mux/1 -> "Valfa/beta "/1
  Vabc/1 -> Fcn1/1, Fcn/1
  Fcn/1 -> Mux/1
  Fcn1/1 -> Mux/2

== system Dfig/Control1/ Angle/abc -> alfa//beta  ==
  Vabc : Inport
  Fcn : Fcn  Expr=2/3*(u[1]-u[2]/2-u[3]/2)
  Fcn1 : Fcn  Expr=2/3*(u[2]*(sqrt(3)/2)-u[3]*(sqrt(3)/2))
  Mux : Mux  Inputs=2
  "Valfa/beta " : Outport
  wires:
  Fcn1/1 -> Mux/2
  Fcn/1 -> Mux/1
  Vabc/1 -> Fcn/1, Fcn1/1
  Mux/1 -> "Valfa/beta "/1
